simulink model "satellite_attitude_determination_and_control"  (R2025b)
settings: Solver=ode4  StartTime=0.0  StopTime=300  FixedStep=0.01  RelTol=1e-3
InitFcn:
  | clear; clc;
  | 
  | Lx = 0.30;Ly = 0.20;Lz = 0.10;
  | m_sat = 10;
  | 
  | Jxx = (1/12) * m_sat * (Ly^2 + Lz^2);Jyy = (1/12) * m_sat * (Lx^2 + Lz^2);Jzz = (1/12) * m_sat * (Lx^2 + Ly^2);
  | 
  | J = diag([Jxx, Jyy, Jzz]);
  | J_inv = inv(J);
  | 
  | A_c = [zeros(3,3), 0.5*eye(3);
  |        zeros(3,3), zeros(3,3)];
  | 
  | B_c = [zeros(3,3);
  |        -J_inv];
  | 
  | C_c = eye(6);
  | D_c = zeros(6,3);
  | 
  | %% LQR CONTROLLER
  | Q = diag([300, 300, 300,30,  30,  30]);
  | R = diag([3, 3, 3]);
  | K = lqr(A_c, B_c, Q, R);
  | %% MPC CONTROLLER
  | Ts = 0.01;
  | sys_continuous = ss(A_c, B_c, C_c, D_c);
  | sys_discrete = c2d(sys_continuous, Ts);
  | mpc_obj = mpc(sys_discrete, Ts);
  | mpc_obj.PredictionHorizon = 10;
  | mpc_obj.ControlHorizon = 2;
  | mpc_obj.Weights.OutputVariables = [300, 300, 300, 30, 30, 30];
  | mpc_obj.Weights.ManipulatedVariables = [3, 3, 3];
  | for i = 1:3
  |     mpc_obj.ManipulatedVariables(i).Min = -0.007;
  |     mpc_obj.ManipulatedVariables(i).Max = 0.007;
  | end
  | 
  | %% Initial Conditions
  | omega_orbit = 0.0011;
  | w0 = [0.002; -omega_orbit + 0.003; -0.001];
  | euler_angles_deg = [12, -15, 10];
  | q0 = eul2quat(deg2rad(euler_angles_deg), "XYZ")';
  | x0_linear = [q0(2); q0(3); q0(4); w0(1); w0(2); w0(3)];
libraries: aerolibutil x2, matrix_library x1, mpclib x1
settings Model: SimulationMode=accelerator  Creator=serha  LastModifiedBy=serha

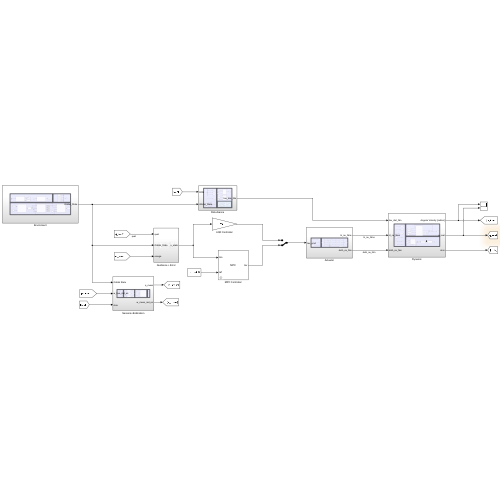
[thumbnail: Simulink's stored preview of the top-level diagram]
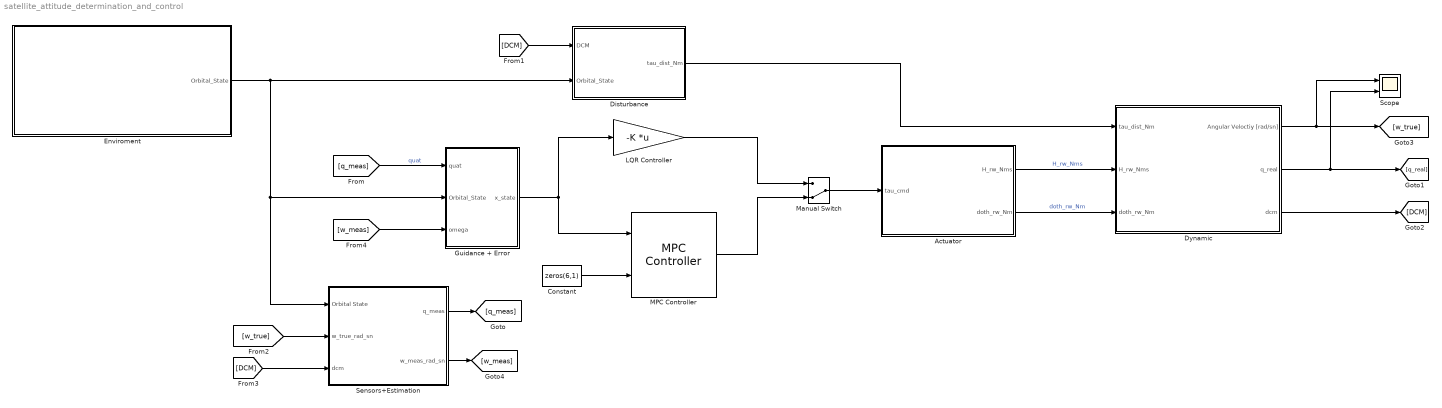
== system satellite_attitude_determination_and_control ==
  Actuator : Subsystem
  Constant : Constant  Value=zeros(6,1)
  Disturbance : Subsystem
  Dynamic : Subsystem
  Enviroment : Subsystem
  Guidance + Error : Subsystem
  LQR Controller : Gain  Gain=-K  Multiplication=Matrix(K*u)
  MPC Controller : mpclib/MPC Controller  SCDEnableBlockLinearizationSpecification=on  mpcobj=mpc_obj  is_multiple=0  enable_value=0  return_u0=off  updateMPCinCallerWorkspace=on  md_inport=off  mv_inport=off  uref_inport=off  return_cost=off  return_mvseq=off  return_qpstatus=off  return_xseq=off  return_state=off  return_ovseq=off  state_inport=off  umin_inport=off  umax_inport=off  ymin_inport=off  ymax_inport=off  cc_inport=off  ywt_inport=off  uwt_inport=off  duwt_inport=off  rhoeps_inport=off  pm_inport=off  MaximumP=10  HorizonChoice=FixedHorizon  n_ts=0.01  n_p=10  n_mv=3  n_md=0  n_ud=0  n_mo=6  n_uo=0  BlockDataType=double  SampleTimeInherited=off  switch_inport=off
  Manual Switch : ManualSwitch  CurrentSetting=0
  Scope : Scope  NumInputPorts=2
      settings: ActiveDisplayYMinimum=-0.67502111832749856  ActiveDisplayYMaximum=1.1081210914767978  DataLoggingVariableName=ScopeData2
  Sensors+Estimation : Subsystem
  wires:
  Actuator/2(doth_rw_Nm) -> Dynamic/3("doth_rw_Nm ")  "doth_rw_Nm"
  Sensors+Estimation/2(w_meas_rad_sn) -> [w_meas]
  [q_meas] -> Guidance + Error/1(quat)  "quat"
  Enviroment/1(Orbital_State) -> Disturbance/2(Orbital_State), Sensors+Estimation/1(Orbital State), Guidance + Error/2(Orbital_State)
  [DCM] -> Disturbance/1(DCM)
  Dynamic/3(dcm) -> [DCM]
  MPC Controller/1 -> Manual Switch/2
  [w_true] -> Sensors+Estimation/2(w_true_rad_sn)
  LQR Controller/1 -> Manual Switch/1
  Sensors+Estimation/1(q_meas) -> [q_meas]
  Actuator/1(H_rw_Nms) -> Dynamic/2(H_rw_Nms)  "H_rw_Nms"
  Manual Switch/1 -> Actuator/1(tau_cmd)
  [w_meas] -> Guidance + Error/3(omega)
  Constant/1 -> MPC Controller/2
  [DCM] -> Sensors+Estimation/3(dcm)
  Disturbance/1(tau_dist_Nm) -> Dynamic/1(tau_dist_Nm)
  Guidance + Error/1(x_state) -> LQR Controller/1, MPC Controller/1
  Dynamic/2(q_real) -> [q_real], Scope/2
  Dynamic/1(Angular Veloctiy [rad/sn]) -> [w_true], Scope/1

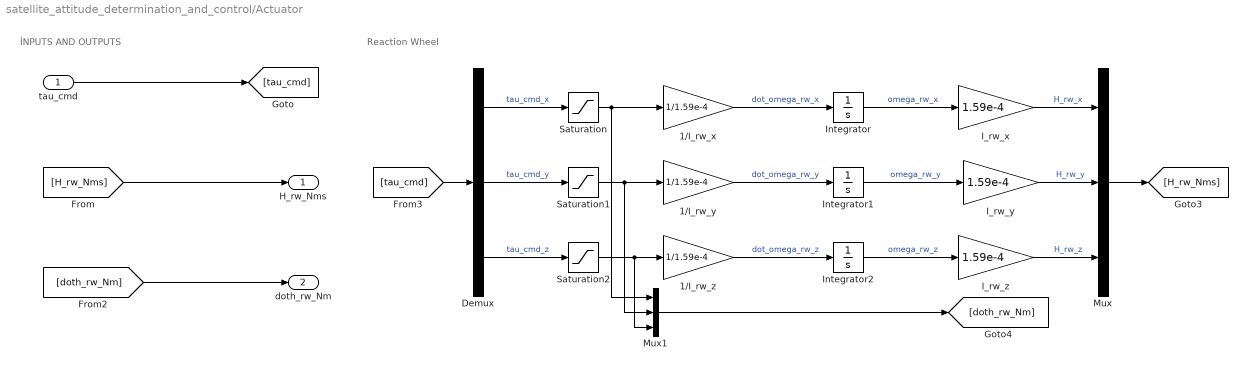
== system satellite_attitude_determination_and_control/Actuator ==
  note: Reaction Wheel
  note: İNPUTS AND OUTPUTS
  tau_cmd : Inport
  1/I_rw_x : Gain  Gain=1/1.59e-4
  1/I_rw_y : Gain  Gain=1/1.59e-4
  1/I_rw_z : Gain  Gain=1/1.59e-4
  Demux : Demux  Outputs=3
  I_rw_x : Gain  Gain=1.59e-4
  I_rw_y : Gain  Gain=1.59e-4
  I_rw_z : Gain  Gain=1.59e-4
  Integrator : Integrator  LimitOutput=on  UpperSaturationLimit=0.1  LowerSaturationLimit=-0.1
  Integrator1 : Integrator  LimitOutput=on  UpperSaturationLimit=0.1  LowerSaturationLimit=-0.1
  Integrator2 : Integrator  LimitOutput=on  UpperSaturationLimit=0.1  LowerSaturationLimit=-0.1
  Mux : Mux  Inputs=3
  Mux1 : Mux  Inputs=3
  Saturation : Saturate  UpperLimit=0.007  LowerLimit=-0.007
  Saturation1 : Saturate  UpperLimit=0.007  LowerLimit=-0.007
  Saturation2 : Saturate  UpperLimit=0.007  LowerLimit=-0.007
  H_rw_Nms : Outport
  doth_rw_Nm : Outport  Port=2
  wires:
  Mux1/1 -> [doth_rw_Nm]
  [tau_cmd] -> Demux/1
  Saturation/1 -> 1/I_rw_x/1, Mux1/1
  1/I_rw_x/1 -> Integrator/1  "dot_omega_rw_x"
  Integrator1/1 -> I_rw_y/1  "omega_rw_y"
  I_rw_x/1 -> Mux/1  "H_rw_x"
  Integrator2/1 -> I_rw_z/1  "omega_rw_z"
  Demux/3 -> Saturation2/1  "tau_cmd_z"
  Demux/1 -> Saturation/1  "tau_cmd_x"
  I_rw_y/1 -> Mux/2  "H_rw_y"
  Saturation1/1 -> 1/I_rw_y/1, Mux1/2
  tau_cmd/1 -> [tau_cmd]
  1/I_rw_z/1 -> Integrator2/1  "dot_omega_rw_z"
  I_rw_z/1 -> Mux/3  "H_rw_z"
  1/I_rw_y/1 -> Integrator1/1  "dot_omega_rw_y"
  [doth_rw_Nm] -> doth_rw_Nm/1
  Saturation2/1 -> 1/I_rw_z/1, Mux1/3
  Integrator/1 -> I_rw_x/1  "omega_rw_x"
  [H_rw_Nms] -> H_rw_Nms/1
  Mux/1 -> [H_rw_Nms]
  Demux/2 -> Saturation1/1  "tau_cmd_y"

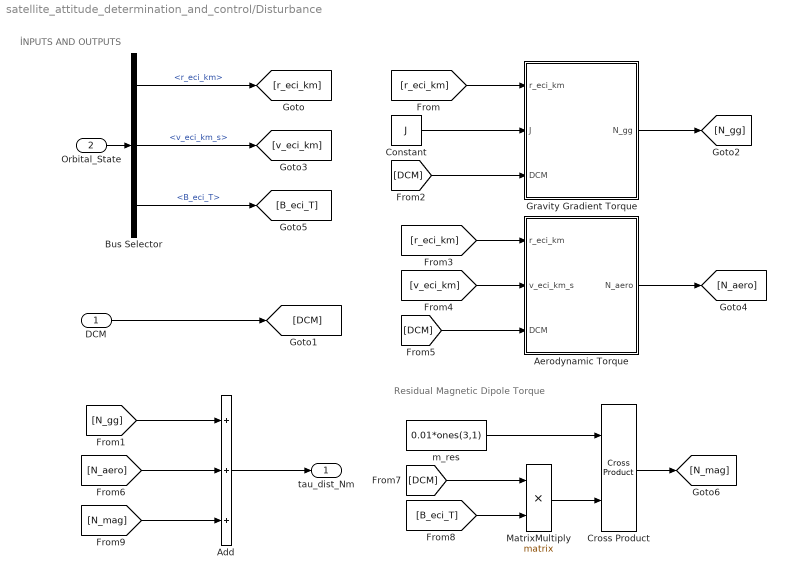
== system satellite_attitude_determination_and_control/Disturbance ==
  note: İNPUTS AND OUTPUTS
  note: Residual Magnetic Dipole Torque
  DCM : Inport
  Orbital_State : Inport  Port=2
  Add : Sum  Inputs=+++
  Aerodynamic Torque : MATLAB Function  TreatAsAtomicUnit=on
  Bus Selector : BusSelector  OutputSignals=r_eci_km,v_eci_km_s,B_eci_T
  Constant : Constant  Value=J
  Cross Product : matrix_library/Cross Product
  Gravity Gradient Torque : MATLAB Function  TreatAsAtomicUnit=on
  MatrixMultiply : Product  Multiplication=Matrix(*)
  m_res : Constant  Value=0.01*ones(3,1)
  tau_dist_Nm : Outport
  wires:
  DCM/1 -> [DCM]
  Constant/1 -> Gravity Gradient Torque/2(J)
  [r_eci_km] -> Gravity Gradient Torque/1(r_eci_km)
  [DCM] -> Gravity Gradient Torque/3(DCM)
  Gravity Gradient Torque/1(N_gg) -> [N_gg]
  [N_gg] -> Add/1
  Add/1 -> tau_dist_Nm/1
  [r_eci_km] -> Aerodynamic Torque/1(r_eci_km)
  [v_eci_km] -> Aerodynamic Torque/2(v_eci_km_s)
  [DCM] -> Aerodynamic Torque/3(DCM)
  Aerodynamic Torque/1(N_aero) -> [N_aero]
  [N_aero] -> Add/2
  [DCM] -> MatrixMultiply/1
  [B_eci_T] -> MatrixMultiply/2
  MatrixMultiply/1 -> Cross Product/2
  m_res/1 -> Cross Product/1
  Cross Product/1 -> [N_mag]
  [N_mag] -> Add/3
  Orbital_State/1 -> Bus Selector/1
  Bus Selector/1 -> [r_eci_km]  "<r_eci_km>"
  Bus Selector/2 -> [v_eci_km]  "<v_eci_km_s>"
  Bus Selector/3 -> [B_eci_T]  "<B_eci_T>"

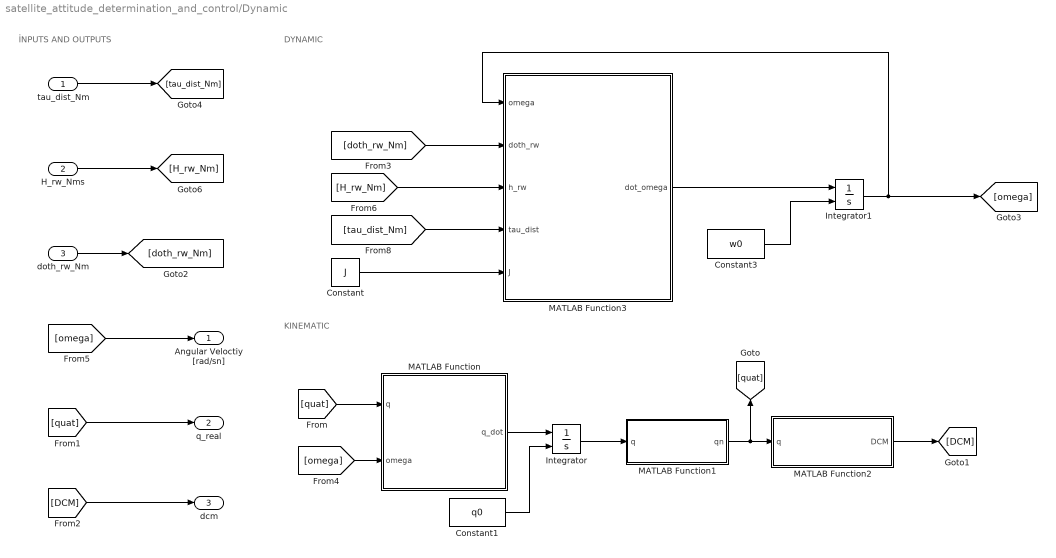
== system satellite_attitude_determination_and_control/Dynamic ==
  note: KINEMATIC
  note: DYNAMIC
  note: İNPUTS AND OUTPUTS
  tau_dist_Nm : Inport
  H_rw_Nms : Inport  Port=2
  "doth_rw_Nm " : Inport  Port=3
  Constant : Constant  Value=J
  Constant1 : Constant  Value=q0
  Constant3 : Constant  Value=w0
  Integrator : Integrator  InitialConditionSource=external  InitialCondition=q0
  Integrator1 : Integrator  InitialConditionSource=external  InitialCondition=w0
  MATLAB Function : MATLAB Function  TreatAsAtomicUnit=on
  MATLAB Function1 : MATLAB Function  TreatAsAtomicUnit=on
  MATLAB Function2 : MATLAB Function  TreatAsAtomicUnit=on
  MATLAB Function3 : MATLAB Function  TreatAsAtomicUnit=on
  Angular Veloctiy [rad/sn] : Outport
  q_real : Outport  Port=2
  dcm : Outport  Port=3
  wires:
  [omega] -> Angular Veloctiy [rad/sn]/1
  [DCM] -> dcm/1
  [doth_rw_Nm] -> MATLAB Function3/2(doth_rw)
  Constant/1 -> MATLAB Function3/5(J)
  Integrator1/1 -> MATLAB Function3/1(omega), [omega]
  MATLAB Function3/1(dot_omega) -> Integrator1/1
  MATLAB Function2/1(DCM) -> [DCM]
  Constant3/1 -> Integrator1/2
  [quat] -> MATLAB Function/1(q)
  Constant1/1 -> Integrator/2
  [quat] -> q_real/1
  [omega] -> MATLAB Function/2(omega)
  Integrator/1 -> MATLAB Function1/1(q)
  MATLAB Function1/1(qn) -> MATLAB Function2/1(q), [quat]
  "doth_rw_Nm "/1 -> [doth_rw_Nm]
  MATLAB Function/1(q_dot) -> Integrator/1
  [H_rw_Nm] -> MATLAB Function3/3(h_rw)
  H_rw_Nms/1 -> [H_rw_Nm]
  [tau_dist_Nm] -> MATLAB Function3/4(tau_dist)
  tau_dist_Nm/1 -> [tau_dist_Nm]

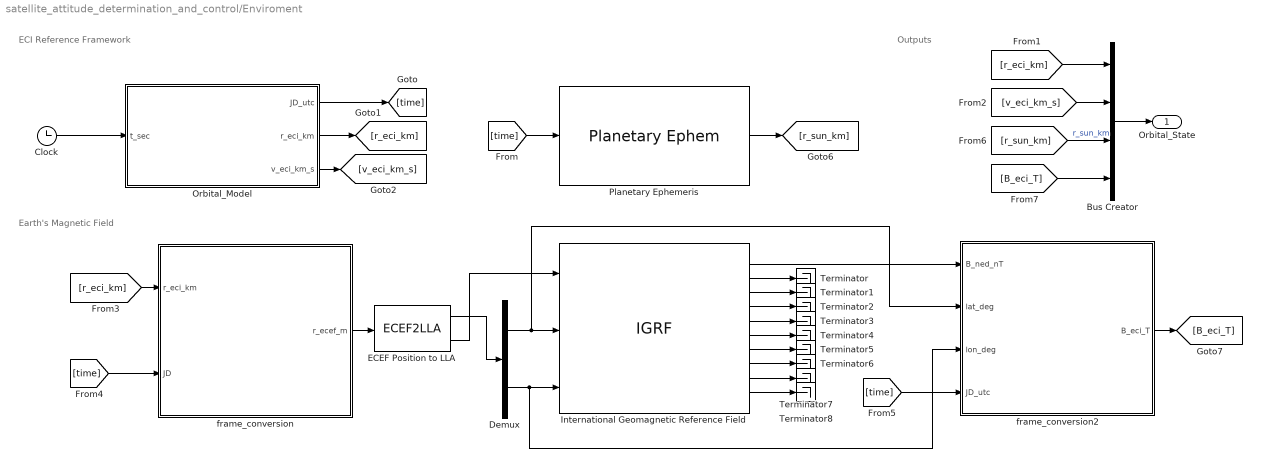
== system satellite_attitude_determination_and_control/Enviroment ==
  note: Outputs
  note: Earth's Magnetic Field
  note: ECI Reference Framework
  Bus Creator : BusCreator  Inputs=4
  Clock : Clock
  Demux : Demux  Outputs=2
  ECEF Position to LLA : ECEF2LLA
  International Geomagnetic Reference Field : IGRF  time_in=off  month=March  day=4  year=2026
      settings: AttributesFormatString=%<generation>
  Orbital_Model : MATLAB Function  TreatAsAtomicUnit=on
  Planetary Ephemeris : PlanetaryEphem  target=Sun  outputVelocity=off
  Terminator{,1..8} (9 alike) : Terminator
  frame_conversion : MATLAB Function  TreatAsAtomicUnit=on
  frame_conversion2 : MATLAB Function  TreatAsAtomicUnit=on
  Orbital_State : Outport
  wires:
  Orbital_Model/2(r_eci_km) -> [r_eci_km]
  Clock/1 -> Orbital_Model/1(t_sec)
  Orbital_Model/1(JD_utc) -> [time]
  Orbital_Model/3(v_eci_km_s) -> [v_eci_km_s]
  [v_eci_km_s] -> Bus Creator/2
  [r_eci_km] -> Bus Creator/1
  Bus Creator/1 -> Orbital_State/1
  [time] -> Planetary Ephemeris/1
  [time] -> frame_conversion/2(JD)
  Demux/2 -> International Geomagnetic Reference Field/3, frame_conversion2/3(lon_deg)
  International Geomagnetic Reference Field/3 -> Terminator1/1
  [time] -> frame_conversion2/4(JD_utc)
  ECEF Position to LLA/1 -> Demux/1
  International Geomagnetic Reference Field/8 -> Terminator6/1
  Planetary Ephemeris/1 -> [r_sun_km]
  frame_conversion/1(r_ecef_m) -> ECEF Position to LLA/1
  International Geomagnetic Reference Field/6 -> Terminator4/1
  International Geomagnetic Reference Field/7 -> Terminator5/1
  International Geomagnetic Reference Field/4 -> Terminator2/1
  Demux/1 -> International Geomagnetic Reference Field/2, frame_conversion2/2(lat_deg)
  [r_eci_km] -> frame_conversion/1(r_eci_km)
  frame_conversion2/1(B_eci_T) -> [B_eci_T]
  International Geomagnetic Reference Field/2 -> Terminator/1
  International Geomagnetic Reference Field/10 -> Terminator8/1
  International Geomagnetic Reference Field/9 -> Terminator7/1
  International Geomagnetic Reference Field/5 -> Terminator3/1
  ECEF Position to LLA/2 -> International Geomagnetic Reference Field/1
  International Geomagnetic Reference Field/1 -> frame_conversion2/1(B_ned_nT)
  [r_sun_km] -> Bus Creator/3  "r_sun_km"
  [B_eci_T] -> Bus Creator/4

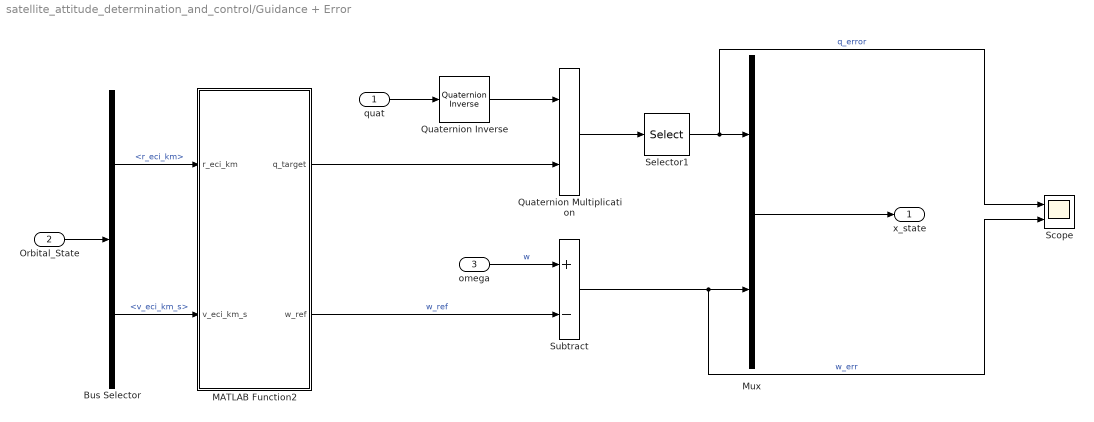
== system satellite_attitude_determination_and_control/Guidance + Error ==
  quat : Inport
  Orbital_State : Inport  Port=2
  omega : Inport  Port=3
  Bus Selector : BusSelector  OutputSignals=r_eci_km,v_eci_km_s
  MATLAB Function2 : MATLAB Function  TreatAsAtomicUnit=on
  Mux : Mux  Inputs=2
  Quaternion Inverse : aerolibutil/Quaternion Inverse
  Quaternion Multiplication : aerolibutil/Quaternion Multiplication
  Scope : Scope  NumInputPorts=2
      settings: ActiveDisplayYMinimum=-0.99192853677037685  ActiveDisplayYMaximum=0.79108806505840579
  Selector1 : Selector  InputPortWidth=4  IndexOptions=Index vector (dialog)  Indices=[2 3 4]  OutputSizes=1
  Subtract : Sum  Inputs=+-
  x_state : Outport
  wires:
  quat/1 -> Quaternion Inverse/1
  MATLAB Function2/1(q_target) -> Quaternion Multiplication/2
  Quaternion Inverse/1 -> Quaternion Multiplication/1
  Mux/1 -> x_state/1
  omega/1 -> Subtract/1  "w"
  MATLAB Function2/2(w_ref) -> Subtract/2  "w_ref"
  Subtract/1 -> Scope/2, Mux/2  "w_err"
  Selector1/1 -> Scope/1, Mux/1  "q_error"
  Orbital_State/1 -> Bus Selector/1
  Bus Selector/1 -> MATLAB Function2/1(r_eci_km)  "<r_eci_km>"
  Bus Selector/2 -> MATLAB Function2/2(v_eci_km_s)  "<v_eci_km_s>"
  Quaternion Multiplication/1 -> Selector1/1

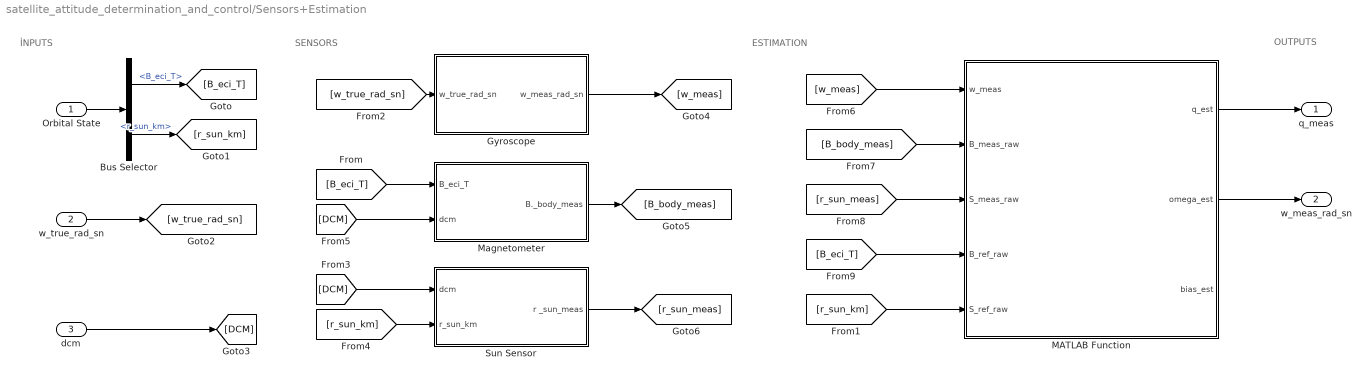
== system satellite_attitude_determination_and_control/Sensors+Estimation ==
  note: OUTPUTS
  note: ESTIMATION
  note: SENSORS
  note: İNPUTS
  Orbital State : Inport
  w_true_rad_sn : Inport  Port=2
  dcm : Inport  Port=3
  Bus Selector : BusSelector  OutputSignals=B_eci_T,r_sun_km
  Gyroscope : Subsystem
  MATLAB Function : MATLAB Function  TreatAsAtomicUnit=on
  Magnetometer : Subsystem
  Sun Sensor : Subsystem
  q_meas : Outport
  w_meas_rad_sn : Outport  Port=2
  wires:
  MATLAB Function/2(omega_est) -> w_meas_rad_sn/1
  Orbital State/1 -> Bus Selector/1
  MATLAB Function/1(q_est) -> q_meas/1
  dcm/1 -> [DCM]
  Bus Selector/2 -> [r_sun_km]  "<r_sun_km>"
  Bus Selector/1 -> [B_eci_T]  "<B_eci_T>"
  w_true_rad_sn/1 -> [w_true_rad_sn]
  [r_sun_km] -> MATLAB Function/5(S_ref_raw)
  [w_true_rad_sn] -> Gyroscope/1(w_true_rad_sn)
  [B_eci_T] -> Magnetometer/1(B_eci_T)
  [DCM] -> Magnetometer/2(dcm)
  [r_sun_km] -> Sun Sensor/2(r_sun_km)
  [DCM] -> Sun Sensor/1(dcm)
  Gyroscope/1(w_meas_rad_sn) -> [w_meas]
  Magnetometer/1(B._body_meas) -> [B_body_meas]
  Sun Sensor/1(r _sun_meas) -> [r_sun_meas]
  [B_body_meas] -> MATLAB Function/2(B_meas_raw)
  [r_sun_meas] -> MATLAB Function/3(S_meas_raw)
  [B_eci_T] -> MATLAB Function/4(B_ref_raw)
  [w_meas] -> MATLAB Function/1(w_meas)

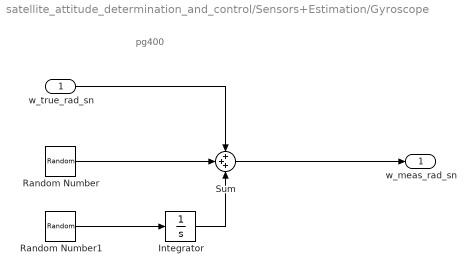
== system satellite_attitude_determination_and_control/Sensors+Estimation/Gyroscope ==
  note: pg400
  w_true_rad_sn : Inport
  Integrator : Integrator  InitialCondition=zeros(3,1)
  Random Number : RandomNumber  Mean=zeros(3,1)  Variance=[4.48e-7 4.48e-7 4.48e-7]'  Seed=[1 2 3]'  SampleTime=0.01
  Random Number1 : RandomNumber  Mean=zeros(3,1)  Variance=[2.35e-13 2.35e-13 2.35e-13]'  Seed=[4 5 6]'  SampleTime=0.01
  Sum : Sum  Inputs=+++
  w_meas_rad_sn : Outport
  wires:
  Random Number1/1 -> Integrator/1
  w_true_rad_sn/1 -> Sum/1
  Random Number/1 -> Sum/2
  Integrator/1 -> Sum/3
  Sum/1 -> w_meas_rad_sn/1

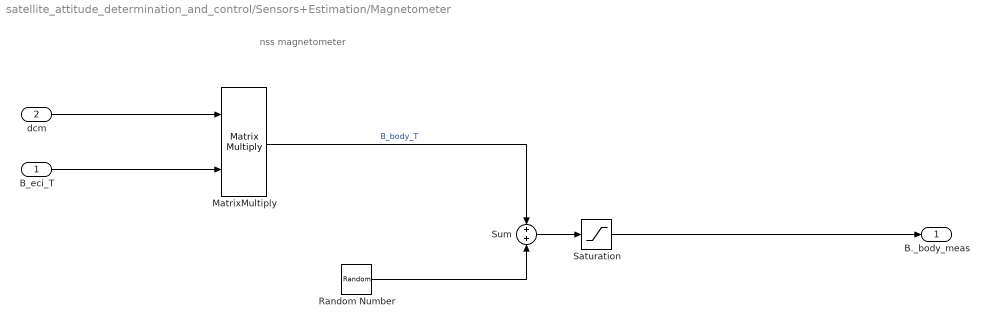
== system satellite_attitude_determination_and_control/Sensors+Estimation/Magnetometer ==
  note: nss magnetometer
  B_eci_T : Inport
  dcm : Inport  Port=2
  MatrixMultiply : Product  Multiplication=Matrix(*)
  Random Number : RandomNumber  Mean=[0 0 0]  Variance=[5.12e-15 5.12e-15 5.12e-15]'  Seed=[7 8 9]'  SampleTime=0.01
  Saturation : Saturate  UpperLimit=6e-5  LowerLimit=-6e-5
  Sum : Sum
  B._body_meas : Outport
  wires:
  dcm/1 -> MatrixMultiply/1
  B_eci_T/1 -> MatrixMultiply/2
  MatrixMultiply/1 -> Sum/1  "B_body_T"
  Sum/1 -> Saturation/1
  Random Number/1 -> Sum/2
  Saturation/1 -> B._body_meas/1

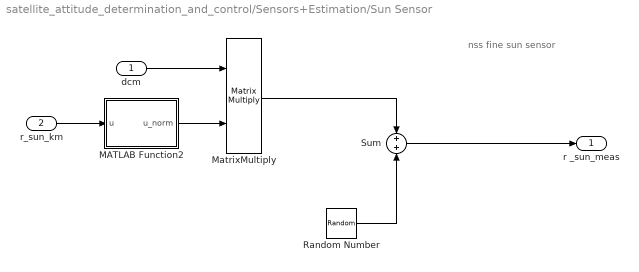
== system satellite_attitude_determination_and_control/Sensors+Estimation/Sun Sensor ==
  note: nss fine sun sensor
  dcm : Inport
  r_sun_km : Inport  Port=2
  MATLAB Function2 : MATLAB Function  TreatAsAtomicUnit=on
  MatrixMultiply : Product  Multiplication=Matrix(*)
  Random Number : RandomNumber  Mean=[0 0 0]'  Variance=[1.218e-5 1.218e-5 1.218e-5]'  Seed=[10 11 12]'  SampleTime=0.01
  Sum : Sum
  r _sun_meas : Outport
  wires:
  dcm/1 -> MatrixMultiply/1
  r_sun_km/1 -> MATLAB Function2/1(u)
  MatrixMultiply/1 -> Sum/1
  Random Number/1 -> Sum/2
  Sum/1 -> r _sun_meas/1
  MATLAB Function2/1(u_norm) -> MatrixMultiply/2

== matlab function satellite_attitude_determination_and_control/Sensors+Estimation/MATLAB Function ==
  settings: updateMethod=DISCRETE
  data: w_meas input; q_est output; B_meas_raw input; S_meas_raw input; B_ref_raw input; S_ref_raw input; omega_est output; bias_est output
function [q_est, omega_est, bias_est] = mekf_estimator(w_meas, B_meas_raw, S_meas_raw, B_ref_raw, S_ref_raw)
dt=0.01;
persistent P q_ref bias_ref is_init
if isempty(is_init)
    q_ref = [1; 0; 0; 0];
    bias_ref = [0; 0; 0];
    P = diag([1e-4, 1e-4, 1e-4, 1e-2, 1e-2, 1e-2]);
    is_init = true;
end
Q_gyro = 4.48e-7 * eye(3);
Q_bias = 2.35e-13 * eye(3);
Q_cont = blkdiag(Q_gyro, Q_bias);
Q_disc = Q_cont * dt;
R_mag = diag([5.12e-15, 5.12e-15, 5.12e-15]);
R_sun = diag([1.218e-5, 1.218e-5, 1.218e-5]);
w_true = w_meas - bias_ref;
wx = w_true(1); wy = w_true(2); wz = w_true(3);
Omega = [ 0, -wx, -wy, -wz;
         wx,  0,  wz, -wy;
         wy, -wz,  0,  wx;
         wz,  wy, -wx,  0];
q_dot = 0.5 * Omega * q_ref;
q_pred = q_ref + q_dot * dt;
q_pred = normalize_quat(q_pred);
bias_pred = bias_ref;
w_skew = skew_sym(w_true);
F = [-w_skew, -eye(3);
    zeros(3,3), zeros(3,3)];
Phi = eye(6) + F * dt;
P_pred = Phi * P * Phi' + Q_disc;
z_mag = norm_vec(B_meas_raw);
ref_mag = norm_vec(B_ref_raw);
A_mat = quaternion_to_dcm(q_pred);
h_mag = A_mat * ref_mag;
y_mag = z_mag - h_mag;
H_mag = [skew_sym(h_mag), zeros(3,3)];
sun_threshold = 1e-3;
if norm(S_meas_raw) > sun_threshold
    z_sun = norm_vec(S_meas_raw);
    ref_sun = norm_vec(S_ref_raw);
    h_sun = A_mat * ref_sun;
    y_sun = z_sun - h_sun;
    H_sun = [skew_sym(h_sun), zeros(3,3)];
    y = [y_mag; y_sun];
    H = [H_mag; H_sun];
    R_current = blkdiag(R_mag, R_sun);
else
    y = y_mag;
    H = H_mag;
    R_current = R_mag;
end
S = H * P_pred * H' + R_current;
K = P_pred * H' / S;
delta_x = K * y;
delta_theta = delta_x(1:3);
delta_bias  = delta_x(4:6);
Xi = [-q_pred(2), -q_pred(3), -q_pred(4);
       q_pred(1), -q_pred(4),  q_pred(3);
       q_pred(4),  q_pred(1), -q_pred(2);
      -q_pred(3),  q_pred(2),  q_pred(1)];
q_ref = q_pred + 0.5 * Xi * delta_theta;
q_ref = normalize_quat(q_ref);
bias_ref = bias_pred + delta_bias;
I = eye(6);
P = (I - K * H) * P_pred * (I - K * H)' + K * R_current * K';
q_est = q_ref;
bias_est = bias_ref;
omega_est = w_meas - bias_est;
end

function S = skew_sym(v)
S = [ 0,     -v(3),  v(2);
      v(3),   0,    -v(1);
     -v(2),   v(1),  0];
end

function qn = normalize_quat(q)
n = norm(q);
if n < 1e-12
    qn = [1;0;0;0];
else
    qn = q / n;
end
end

function vn = norm_vec(v)
n = norm(v);
if n < 1e-12
    vn = [0;0;0];
else
    vn = v / n;
end
end

function DCM = quaternion_to_dcm(q)
q0 = q(1); q1 = q(2); q2 = q(3); q3 = q(4);
DCM = [1 - 2*(q2^2 + q3^2),   2*(q1*q2 + q0*q3),   2*(q1*q3 - q0*q2);
       2*(q1*q2 - q0*q3),     1 - 2*(q1^2 + q3^2), 2*(q2*q3 + q0*q1);
       2*(q1*q3 + q0*q2),     2*(q2*q3 - q0*q1),   1 - 2*(q1^2 + q2^2)];
end

== matlab function satellite_attitude_determination_and_control/Sensors+Estimation/Sun Sensor/MATLAB Function2 ==
  data: u input; u_norm output
function u_norm = normalize_vector(u)
    % u: 3x1 boyutunda giriş vektörü (Manyetik alan veya Güneş vektörü)
    
    % Vektörün normunu (büyüklüğünü) hesapla
    v_norm = norm(u);
    
    % Sıfıra bölünme hatasını engellemek için küçük bir tolerans (1e-12) ekle
    if v_norm < 1e-12
        u_norm = [0; 0; 0]; % Eğer vektör tamamen sıfırsa, sıfır vektörü döndür
    else
        u_norm = u / v_norm; % Gerçek birim vektör işlemi (u / ||u||)
    end
end

== matlab function satellite_attitude_determination_and_control/Disturbance/Aerodynamic Torque ==
  data: r_eci_km input; N_aero output; v_eci_km_s input; DCM input
function N_aero  = aero_torque(r_eci_km, v_eci_km_s, DCM)
wE = [0; 0; 7.2921150e-5];
Re = 6378137;
Cd = 2.2;
Lx = 0.30;
Ly = 0.20;
Lz = 0.10;
Ax = Ly * Lz;
Ay = Lx * Lz;
Az = Lx * Ly;
r_cp = [0.005; -0.003; 0.002];
r_eci_km   = r_eci_km(:);
v_eci_km_s = v_eci_km_s(:);
r_eci = 1000 * r_eci_km;
v_eci = 1000 * v_eci_km_s;
r = norm(r_eci);
h = r - Re;
h_ref   = 400e3;
rho_ref = 4e-12;
H       = 50e3;
rho = rho_ref * exp(-(h - h_ref)/H);
if rho < 1e-15
    rho = 1e-15;
elseif rho > 1e-9
    rho = 1e-9;
end
v_rel_eci = v_eci - cross(wE, r_eci);
v_rel_b   = DCM * v_rel_eci;
V = norm(v_rel_b);
if V < 1e-9
    N_aero = [0;0;0];
    A_eff = 0;
    return;
end
v_hat_b = v_rel_b / V;
A_eff = Ax * abs(v_hat_b(1)) + ...
        Ay * abs(v_hat_b(2)) + ...
        Az * abs(v_hat_b(3));
F_aero_b = -0.5 * rho * V^2 * Cd * A_eff * v_hat_b;
N_aero = cross(r_cp, F_aero_b);
end

== matlab function satellite_attitude_determination_and_control/Dynamic/MATLAB Function ==
  data: q input; q_dot output; omega input
function q_dot = quaternion_kinematic(q, omega)
wx = omega(1);wy = omega(2);wz = omega(3);
Omega=[0,-wx,-wy,-wz;
       wx,0,wz,-wy;
       wy,-wz,0,wx;
       wz,wy,-wx,0];
q_dot=0.5*Omega*q;
end

== matlab function satellite_attitude_determination_and_control/Dynamic/MATLAB Function1 ==
  data: q input; qn output
function qn = normalize_quaternion(q)
n = norm(q);
if n < 1e-12
    qn = [1;0;0;0];
else
    qn = q / n;
end
end

== matlab function satellite_attitude_determination_and_control/Dynamic/MATLAB Function2 ==
  data: q input; DCM output
function DCM = quaternion_to_dcm(q)
q0 = q(1);q1 = q(2);q2 = q(3);q3 = q(4);

DCM = [1 - 2*(q2^2 + q3^2),   2*(q1*q2 + q0*q3),   2*(q1*q3 - q0*q2);
       2*(q1*q2 - q0*q3),     1 - 2*(q1^2 + q3^2), 2*(q2*q3 + q0*q1);
       2*(q1*q3 + q0*q2),     2*(q2*q3 - q0*q1),   1 - 2*(q1^2 + q2^2)];
end

== matlab function satellite_attitude_determination_and_control/Enviroment/frame_conversion ==
  data: r_eci_km input; r_ecef_m output; JD input
function r_ecef_m = ECI2ECEF(r_eci_km, JD)
r_eci = 1000 * r_eci_km;
T = (JD - 2451545.0)/36525;
theta = 280.46061837 ...
      + 360.98564736629*(JD - 2451545.0) ...
      + 0.000387933*T*T ...
      - (T^3)/38710000;
theta = mod(theta,360);
theta = deg2rad(theta);
c = cos(theta);
s = sin(theta);
R = [ c -s 0;
      s  c 0;
      0  0 1];
r_ecef_m = R * r_eci;
end

== matlab function satellite_attitude_determination_and_control/Dynamic/MATLAB Function3 ==
  data: omega input; doth_rw input; h_rw input; tau_dist input; dot_omega output; J input
function dot_omega = dynamic(omega, doth_rw, h_rw, tau_dist, J)
%#codegen

dot_omega = J \ ( tau_dist - doth_rw - cross(omega, J*omega + h_rw));

== matlab function satellite_attitude_determination_and_control/Enviroment/Orbital_Model ==
  data: t_sec input; JD_utc output; r_eci_km output; v_eci_km_s output
function [JD_utc, r_eci_km, v_eci_km_s] = orbital(t_sec)
mu = 398600.4418; % [km^3/s^2]
JD_epoch = 2461103.68048341;
JD_utc = JD_epoch + t_sec/86400.0;
e        = 0.0000486;
i    = deg2rad(97.3829);
raan = deg2rad(141.2763);
argp = deg2rad(320.0226);
M0   = deg2rad(40.0975);
n_revday = 15.22843827;
n = n_revday * 2*pi / 86400.0;
a = (mu/(n*n))^(1/3);
M = M0 + n*t_sec;
M = wrapToPi_codegen(M);
E = kepler_E_newton(M, e);
nu = 2*atan2( sqrt(1+e)*sin(0.5*E), sqrt(1-e)*cos(0.5*E) );
p = a*(1 - e*e);
r = p/(1 + e*cos(nu));
r_pqw = [r*cos(nu); r*sin(nu); 0];
v_pqw = sqrt(mu/p) * [-sin(nu); e + cos(nu); 0];
Q = R3(raan) * R1(i) * R3(argp);
r_eci_km  = Q * r_pqw;
v_eci_km_s = Q * v_pqw;
end

function E = kepler_E_newton(M, e)
E = M;
for k = 1:30
    f  = E - e*sin(E) - M;
    fp = 1 - e*cos(E);
    dE = -f/fp;
    E  = E + dE;
    if abs(dE) < 1e-12
        break;
    end
end
end

function y = wrapToPi_codegen(x)
y = mod(x + pi, 2*pi) - pi;
end

function A = R1(th)
c = cos(th); s = sin(th);
A = [1 0 0;
     0 c -s;
     0 s  c];
end

function A = R3(th)
c = cos(th); s = sin(th);
A = [ c -s 0;
      s  c 0;
      0  0 1];
end

== matlab function satellite_attitude_determination_and_control/Guidance + Error/MATLAB Function2 ==
  data: r_eci_km input; q_target output; v_eci_km_s input; w_ref output
function [q_target, w_ref] = nadir_target_from_orbit(r_eci_km, v_eci_km_s)
z_ref = -r_eci_km / norm(r_eci_km);
h_eci = cross(r_eci_km, v_eci_km_s);
y_ref = -h_eci / norm(h_eci);
x_ref = cross(y_ref, z_ref);
x_ref = x_ref / norm(x_ref);
y_ref = cross(z_ref, x_ref);
y_ref = y_ref / norm(y_ref);
C_ref_to_eci = [x_ref, y_ref, z_ref];
C_eci_to_ref = C_ref_to_eci';
q_target_row = rotm2quat(C_eci_to_ref);
q_target = q_target_row(:);
w_ref_eci = h_eci / (norm(r_eci_km)^2);
w_ref = C_eci_to_ref * w_ref_eci;

== matlab function satellite_attitude_determination_and_control/Enviroment/frame_conversion2 ==
  data: B_ned_nT input; B_eci_T output; lat_deg input; lon_deg input; JD_utc input
function B_eci_T = IGRF_NED_to_ECI_Tesla(B_ned_nT, lat_deg, lon_deg, JD_utc)
B_ned_T = 1e-9 * B_ned_nT;
deg = pi/180;
phi = lat_deg*deg;
lam = lon_deg*deg;
sphi = sin(phi); cphi = cos(phi);
slam = sin(lam); clam = cos(lam);
R_ned2ecef = [ -sphi*clam,  -slam,  -cphi*clam;
              -sphi*slam,   clam,  -cphi*slam;
               cphi,        0,     -sphi      ];
B_ecef_T = R_ned2ecef * B_ned_T;
theta = gmst_rad(JD_utc);
c = cos(theta); s = sin(theta);
R_ecef2eci = [ c, -s, 0;
               s,  c, 0;
               0,  0, 1];
B_eci_T = R_ecef2eci * B_ecef_T;
end

function theta = gmst_rad(JD)
T = (JD - 2451545.0)/36525.0;
theta_deg = 280.46061837 ...
          + 360.98564736629*(JD - 2451545.0) ...
          + 0.000387933*T*T ...
          - (T*T*T)/38710000.0;
theta_deg = mod(theta_deg, 360.0);
theta = theta_deg*pi/180.0;
end

== matlab function satellite_attitude_determination_and_control/Disturbance/Gravity Gradient Torque ==
  data: r_eci_km input; N_gg output; J input; DCM input
function N_gg = gg_torque(r_eci_km,J,DCM)
mu = 3.986004418e14;
r_eci=1000 * r_eci_km;
r = norm(r_eci);
r_hat_eci = r_eci / r;
r_hat_b = DCM * r_hat_eci;
N_gg = 3*mu/(r^3) * cross(r_hat_b, J*r_hat_b);
end
